simulink model "cube0_mpcpd_model"  (R2022b)
settings: Solver=VariableStepAuto  StartTime=0.0  StopTime=400  RelTol=1e-3  AbsTol=1e-3
undefined symbols (not defined in the file or in its folder): ks, lambdas
settings Model: Creator=Abhijit  LastModifiedBy=abhij
settings SolverCC: AutoScaleAbsTol=off  AlgebraicLoopSolver=TrustRegion  MaxZcPerStep=1
settings DataIOCC: SaveState=on  StateSaveName=states
settings DebuggingCC: UnconnectedInputMsg=warning  UnconnectedOutputMsg=warning  UnconnectedLineMsg=warning  SymbolicDimsDataTypeCodeGenerationDiagnostic=none  SFMachineParentedDataDiag=warning
settings ModelReferenceCC: EnableRefExpFcnMdlSchedulingChecks=on
settings SFSimCC: CustomCodeUndefinedFunction=UseInterfaceOnly
settings RTWCC: DLArmComputeVersion=19.05
settings SimscapeCC: SimscapeLogType=all  SimscapeLogSimulationStatistics=on  SimscapeLogDataHistory=10000

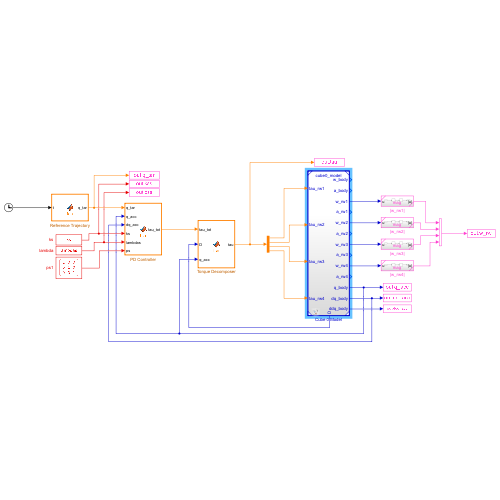
[thumbnail: Simulink's stored preview of the top-level diagram]
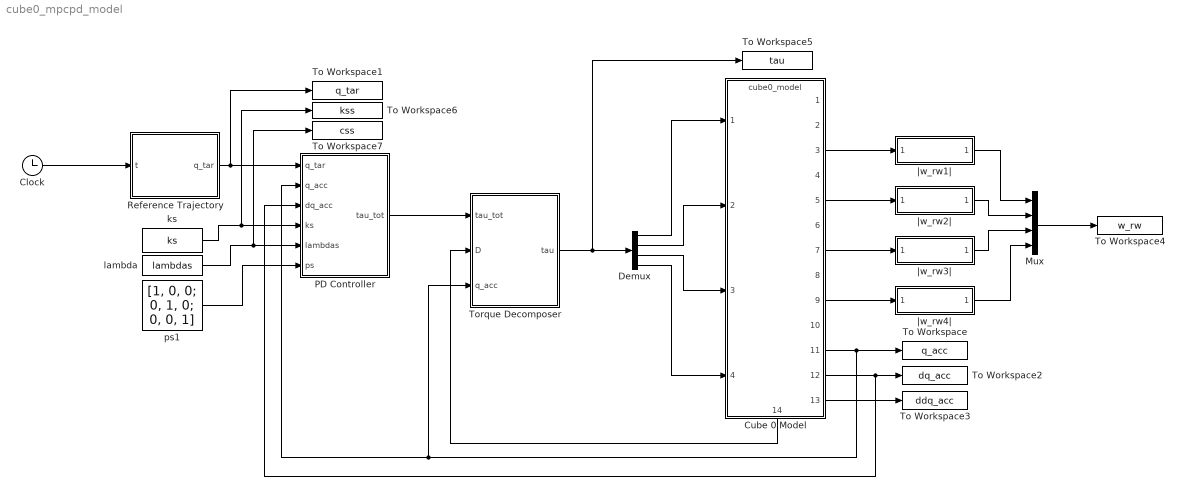
== system cube0_mpcpd_model ==
  Clock : Clock
  Cube 0 Model : ModelReference  ModelNameDialog=cube0_model  SimulationMode=Normal  ModelReferenceVersion=1.24
      settings: PortSchema="{\"entries\":[{\"content\":{\"sides\":[{\"content\":{\"connectorIds\":[\"In1\",\"In2\",\"In3\",\"In4\"]},\"type\":\"ConnectorPlacement.EquallySpacedRectSide\",\"uuid\":\"36a9c944-f213-4c4e-b6f2-fa7d728627b0\"},{\"content\":{\"connectorIds\":[\"Out1\",\"Out2\",\"Out3\",\"Out4\",\"Out5\",\"Out6\",\"Out7\",\"Out8\",\"Out9\",\"Out10\",\"Out11\",\"Out12\",\"Out13\"],\"side\":\"RIGHT\"},\"type\":\"ConnectorPlacement.EquallySpacedRectSide\",\"uuid\":\"ad793041-f32f-405f-9966-9455be290c1c\"},{\"content\":{\"connectorIds\":[],\"side\":\"TOP\"},\"type\":\"ConnectorPlacement.EquallySpacedRectSide\",\"uuid\":\"a8d37d27-2c3a-480b-9200-d310321df053\"},{\"content\":{\"connectorIds\":[\"Out14\"],\"side\":\"BOTTOM\"},\"type\":\"ConnectorPlacement.EquallySpacedRectSide\",\"uuid\":\"c14ee11a-abeb-4912-9eb4-a36323cd54f1\"}]},\"type\":\"ConnectorPlacement.EquallySpacedConnector\",\"uuid\":\"5842ca05-faf4-4c84-934b-15246120a6a0\"}],\"packageUris\":[\"http://schema.mathworks.com/mf0/Connector/R2020b\"],\"version\":\"1.0\"}"
  Demux : Demux
  Mux : Mux
  PD Controller : MATLAB Function  TreatAsAtomicUnit=on
  Reference Trajectory : MATLAB Function  TreatAsAtomicUnit=on
  To Workspace : ToWorkspace  VariableName=q_acc  SaveFormat=Timeseries  SampleTime=-1
  To Workspace1 : ToWorkspace  VariableName=q_tar  SaveFormat=Timeseries  SampleTime=-1
  To Workspace2 : ToWorkspace  VariableName=dq_acc  SaveFormat=Timeseries  SampleTime=-1
  To Workspace3 : ToWorkspace  VariableName=ddq_acc  SaveFormat=Timeseries  SampleTime=-1
  To Workspace4 : ToWorkspace  VariableName=w_rw  SaveFormat=Timeseries  SampleTime=-1
  To Workspace5 : ToWorkspace  VariableName=tau  SaveFormat=Timeseries  SampleTime=-1
  To Workspace6 : ToWorkspace  VariableName=kss  SaveFormat=Timeseries  SampleTime=-1
  To Workspace7 : ToWorkspace  VariableName=css  SaveFormat=Timeseries  SampleTime=-1
  Torque Decomposer : MATLAB Function  TreatAsAtomicUnit=on
  ks : Constant  Value=ks
  lambda : Constant  Value=lambdas
  ps1 : Constant  Value=[1, 0, 0; 0, 1, 0; 0, 0, 1]
  |w_rw1| : Subsystem  ReferencedSubsystem=mag
  |w_rw2| : Subsystem  ReferencedSubsystem=mag
  |w_rw3| : Subsystem  ReferencedSubsystem=mag
  |w_rw4| : Subsystem  ReferencedSubsystem=mag
  wires:
  Cube 0 Model/12 -> To Workspace2/1, PD Controller/3(dq_acc)
  Demux/2 -> Cube 0 Model/2
  ps1/1 -> PD Controller/6(ps)
  Clock/1 -> Reference Trajectory/1(t)
  Demux/3 -> Cube 0 Model/3
  Demux/4 -> Cube 0 Model/4
  Demux/1 -> Cube 0 Model/1
  Torque Decomposer/1(tau) -> To Workspace5/1, Demux/1
  Reference Trajectory/1(q_tar) -> To Workspace1/1, PD Controller/1(q_tar)
  Cube 0 Model/14 -> Torque Decomposer/2(D)
  Cube 0 Model/11 -> To Workspace/1, PD Controller/2(q_acc), Torque Decomposer/3(q_acc)
  PD Controller/1(tau_tot) -> Torque Decomposer/1(tau_tot)
  ks/1 -> To Workspace6/1, PD Controller/4(ks)
  lambda/1 -> To Workspace7/1, PD Controller/5(lambdas)
  Cube 0 Model/5 -> |w_rw2|/1
  Cube 0 Model/9 -> |w_rw4|/1
  |w_rw1|/1 -> Mux/1
  |w_rw3|/1 -> Mux/3
  |w_rw4|/1 -> Mux/4
  Mux/1 -> To Workspace4/1
  Cube 0 Model/7 -> |w_rw3|/1
  Cube 0 Model/13 -> To Workspace3/1
  Cube 0 Model/3 -> |w_rw1|/1
  |w_rw2|/1 -> Mux/2

== matlab function cube0_mpcpd_model/PD Controller ==
  data: tau_tot output; q_tar input; q_acc input; dq_acc input; ks input; lambdas input; ps input
function tau_tot = fcn(q_tar, q_acc, dq_acc, ks, lambdas, ps)
    tau_tot = pdcontroller(q_tar, q_acc, dq_acc, ks, lambdas, ps);

== matlab function cube0_mpcpd_model/Reference Trajectory ==
  settings: updateMethod=CONTINUOUS
  data: t input; q_tar output
function q_tar = fcn(t)
     q_tar = refpath(t, 1);
end

== matlab function cube0_mpcpd_model/Torque Decomposer ==
  data: tau_tot input; tau output; D input; q_acc input
function tau = fcn(tau_tot, D, q_acc)
    tau = taudecomp(tau_tot, D, q_acc);
end
